simulink model "DC_drives_system"  (R2025b)
settings: Solver=FixedStepAuto  StartTime=0.0  StopTime=3.0  FixedStep=1e-4  RelTol=1e-3
values from neighbouring files (symbols this model uses):
  J_load = Simulink.Parameter    [dc_drives_system_parameter_declaraction.m]
  J_motor = Simulink.Parameter    [dc_drives_system_parameter_declaraction.m]    (also in motorised_BoB_system_with_PID.m)
  k_e = Simulink.Parameter    [dc_drives_system_parameter_declaraction.m]    (also in motorised_BoB_system_with_PID.m)
  k_t = Simulink.Parameter    [dc_drives_system_parameter_declaraction.m]    (also in motorised_BoB_system_with_PID.m)
  kFrs = Simulink.Parameter    [dc_drives_system_parameter_declaraction.m]    (also in motorised_BoB_system_with_PID.m)
  L_a = Simulink.Parameter    [dc_drives_system_parameter_declaraction.m]    (also in motorised_BoB_system_with_PID.m)
  R_a = Simulink.Parameter    [dc_drives_system_parameter_declaraction.m]    (also in motorised_BoB_system_with_PID.m)
  t_inv = Simulink.Parameter    [dc_drives_system_parameter_declaraction.m]    (also in motorised_BoB_system_with_PID.m)
  U_DC = Simulink.Parameter    [dc_drives_system_parameter_declaraction.m]    (also in motorised_BoB_system_with_PID.m)
  W_ci = Simulink.Parameter    [dc_drives_system_parameter_declaraction.m]    (also in motorised_BoB_system_with_PID.m)
  W_cq = Simulink.Parameter    [dc_drives_system_parameter_declaraction.m]    (also in motorised_BoB_system_with_PID.m)
  W_cw = Simulink.Parameter    [dc_drives_system_parameter_declaraction.m]    (also in motorised_BoB_system_with_PID.m)
undefined symbols (not defined in the file or in its folder): L, R
settings Model: Creator=fycce  LastModifiedBy=fycce

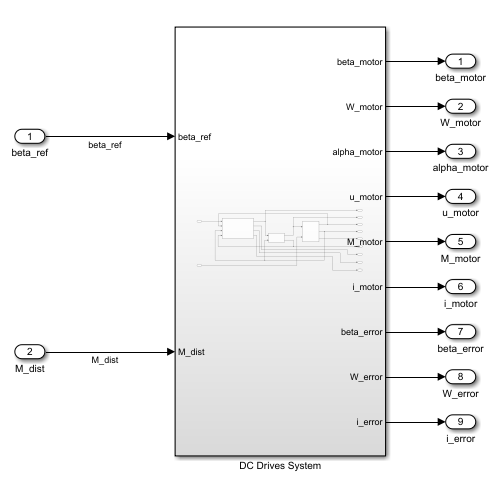
[thumbnail: Simulink's stored preview of the top-level diagram]
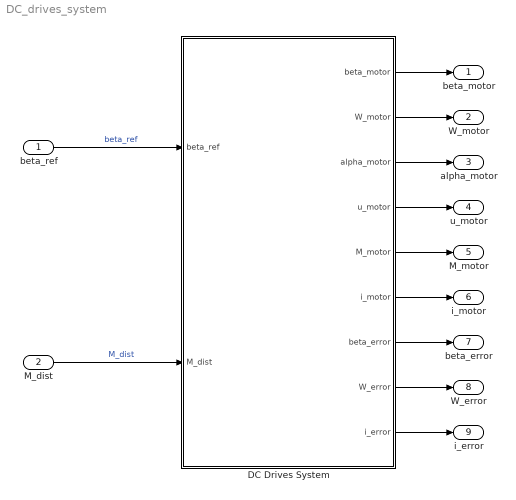
== system DC_drives_system ==
  beta_ref : Inport
  M_dist : Inport  Port=2
  DC Drives System : Subsystem
  beta_motor : Outport
  W_motor : Outport  Port=2
  alpha_motor : Outport  Port=3
  u_motor : Outport  Port=4
  M_motor : Outport  Port=5
  i_motor : Outport  Port=6
  beta_error : Outport  Port=7
  W_error : Outport  Port=8
  i_error : Outport  Port=9
  wires:
  DC Drives System/1(beta_motor) -> beta_motor/1
  DC Drives System/2(W_motor) -> W_motor/1
  DC Drives System/3(alpha_motor) -> alpha_motor/1
  DC Drives System/4(u_motor) -> u_motor/1
  DC Drives System/5(M_motor) -> M_motor/1
  DC Drives System/6(i_motor) -> i_motor/1
  DC Drives System/7(beta_error) -> beta_error/1
  DC Drives System/8(W_error) -> W_error/1
  DC Drives System/9(i_error) -> i_error/1
  M_dist/1 -> DC Drives System/2(M_dist)  "M_dist"
  beta_ref/1 -> DC Drives System/1(beta_ref)  "beta_ref"

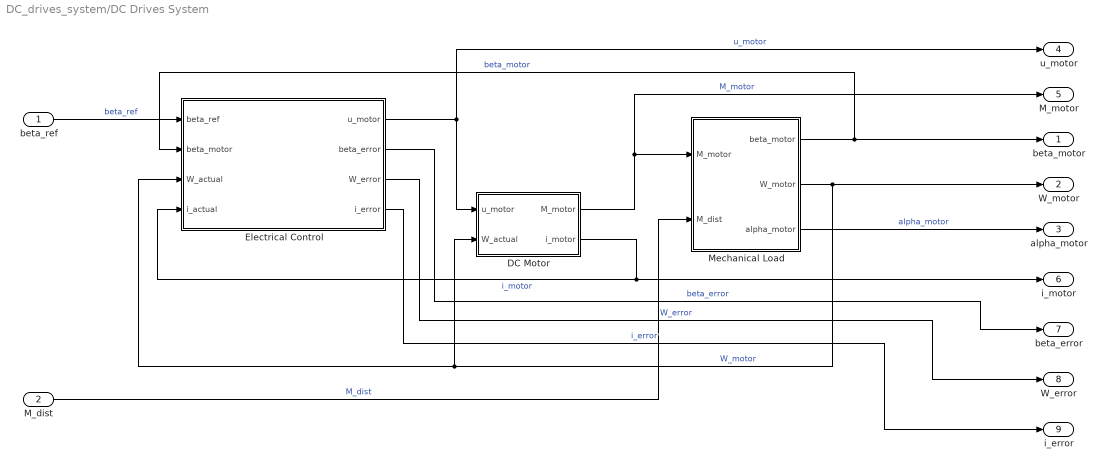
== system DC_drives_system/DC Drives System ==
  beta_ref : Inport
  M_dist : Inport  Port=2
  DC Motor : Subsystem
  Electrical Control : Subsystem
  Mechanical Load : Subsystem
  beta_motor : Outport
  W_motor : Outport  Port=2
  alpha_motor : Outport  Port=3
  u_motor : Outport  Port=4
  M_motor : Outport  Port=5
  i_motor : Outport  Port=6
  beta_error : Outport  Port=7
  W_error : Outport  Port=8
  i_error : Outport  Port=9
  wires:
  Electrical Control/2(beta_error) -> beta_error/1  "beta_error"
  Electrical Control/1(u_motor) -> u_motor/1, DC Motor/1(u_motor)  "u_motor"
  DC Motor/2(i_motor) -> Electrical Control/4(i_actual), i_motor/1  "i_motor"
  Mechanical Load/1(beta_motor) -> beta_motor/1, Electrical Control/2(beta_motor)  "beta_motor"
  Electrical Control/3(W_error) -> W_error/1  "W_error"
  beta_ref/1 -> Electrical Control/1(beta_ref)  "beta_ref"
  Mechanical Load/2(W_motor) -> W_motor/1, DC Motor/2(W_actual), Electrical Control/3(W_actual)  "W_motor"
  DC Motor/1(M_motor) -> M_motor/1, Mechanical Load/1(M_motor)  "M_motor"
  Electrical Control/4(i_error) -> i_error/1  "i_error"
  Mechanical Load/3(alpha_motor) -> alpha_motor/1  "alpha_motor"
  M_dist/1 -> Mechanical Load/2(M_dist)  "M_dist"

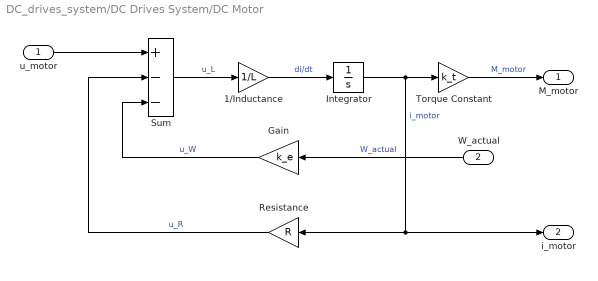
== system DC_drives_system/DC Drives System/DC Motor ==
  u_motor : Inport
  W_actual : Inport  Port=2
  1/Inductance : Gain  Gain=1/L
  Gain : Gain  Gain=k_e
  Integrator : Integrator
  Resistance : Gain  Gain=R
  Sum : Sum  Inputs=+--
  Torque Constant : Gain  Gain=k_t
  M_motor : Outport
  i_motor : Outport  Port=2
  wires:
  u_motor/1 -> Sum/1
  Sum/1 -> 1/Inductance/1  "u_L"
  1/Inductance/1 -> Integrator/1  "di/dt"
  Integrator/1 -> i_motor/1, Resistance/1, Torque Constant/1  "i_motor"
  Torque Constant/1 -> M_motor/1  "M_motor"
  Resistance/1 -> Sum/2  "u_R"
  Gain/1 -> Sum/3  "u_W"
  W_actual/1 -> Gain/1  "W_actual"

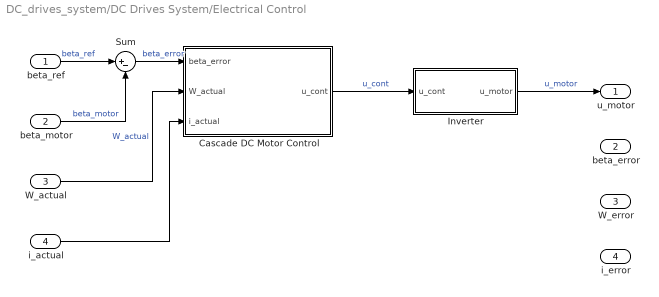
== system DC_drives_system/DC Drives System/Electrical Control ==
  beta_ref : Inport
  beta_motor : Inport  Port=2
  W_actual : Inport  Port=3
  i_actual : Inport  Port=4
  Cascade DC Motor Control : Subsystem
  Inverter : Subsystem
  Sum : Sum  Inputs=|+-
  u_motor : Outport
  beta_error : Outport  Port=2
  W_error : Outport  Port=3
  i_error : Outport  Port=4
  wires:
  Inverter/1(u_motor) -> u_motor/1  "u_motor"
  Cascade DC Motor Control/1(u_cont) -> Inverter/1(u_cont)  "u_cont"
  beta_ref/1 -> Sum/1  "beta_ref"
  beta_motor/1 -> Sum/2  "beta_motor"
  Sum/1 -> Cascade DC Motor Control/1(beta_error)  "beta_error"
  W_actual/1 -> Cascade DC Motor Control/2(W_actual)  "W_actual"
  i_actual/1 -> Cascade DC Motor Control/3(i_actual)

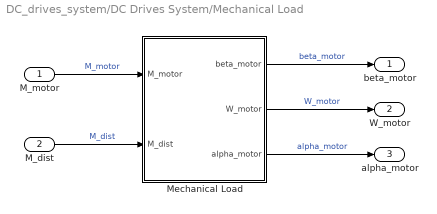
== system DC_drives_system/DC Drives System/Mechanical Load ==
  M_motor : Inport
  M_dist : Inport  Port=2
  Mechanical Load : Subsystem  Variant=on
  beta_motor : Outport
  W_motor : Outport  Port=2
  alpha_motor : Outport  Port=3
  wires:
  M_motor/1 -> Mechanical Load/1(M_motor)  "M_motor"
  Mechanical Load/2(W_motor) -> W_motor/1  "W_motor"
  Mechanical Load/1(beta_motor) -> beta_motor/1  "beta_motor"
  Mechanical Load/3(alpha_motor) -> alpha_motor/1  "alpha_motor"
  M_dist/1 -> Mechanical Load/2(M_dist)  "M_dist"

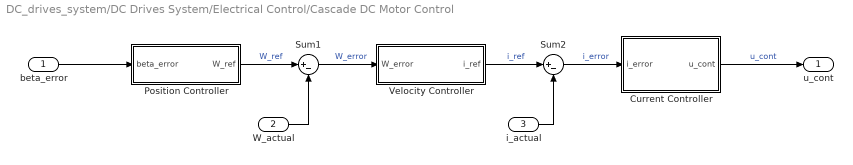
== system DC_drives_system/DC Drives System/Electrical Control/Cascade DC Motor Control ==
  beta_error : Inport
  W_actual : Inport  Port=2
  i_actual : Inport  Port=3
  Current Controller : Subsystem
  Position Controller : Subsystem
  Sum1 : Sum  Inputs=|+-
  Sum2 : Sum  Inputs=|+-
  Velocity Controller : Subsystem
  u_cont : Outport
  wires:
  Position Controller/1(W_ref) -> Sum1/1  "W_ref"
  Sum1/1 -> Velocity Controller/1(W_error)  "W_error"
  Velocity Controller/1(i_ref) -> Sum2/1  "i_ref"
  Sum2/1 -> Current Controller/1(i_error)  "i_error"
  beta_error/1 -> Position Controller/1(beta_error)
  Current Controller/1(u_cont) -> u_cont/1  "u_cont"
  i_actual/1 -> Sum2/2
  W_actual/1 -> Sum1/2

== system DC_drives_system/DC Drives System/Electrical Control/Inverter ==
  u_cont : Inport
  1st Order Lag : Subsystem
  U_DC Saturation : Saturate  UpperLimit=U_DC  LowerLimit=-U_DC
  u_motor : Outport
  wires:
  U_DC Saturation/1 -> u_motor/1  "u_motor"
  u_cont/1 -> 1st Order Lag/1(u_cont)  "u_cont"
  1st Order Lag/1(u_cont_lag) -> U_DC Saturation/1  "u_cont_lag"

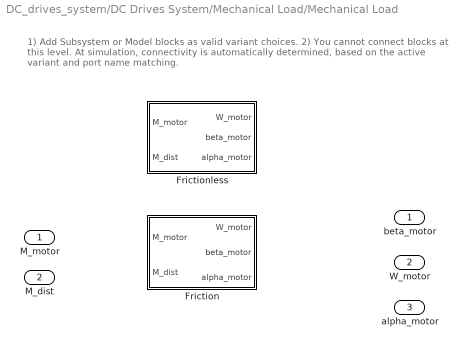
== system DC_drives_system/DC Drives System/Mechanical Load/Mechanical Load ==
  note: 1) Add Subsystem or Model blocks as valid variant choices.
      | 2) You cannot connect blocks at this level. At simulation, connectivity is automatically
      | determined, based on the active variant and port name matching.
  M_motor : Inport
  M_dist : Inport  Port=2
  Friction : Subsystem  VariantControl=choice == 1
  Frictionless : Subsystem  VariantControl=choice == 2
  beta_motor : Outport
  W_motor : Outport  Port=2
  alpha_motor : Outport  Port=3

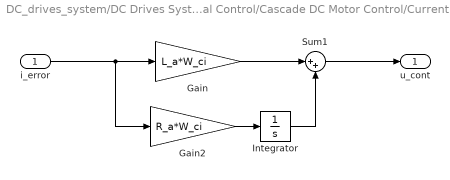
== system DC_drives_system/DC Drives System/Electrical Control/Cascade DC Motor Control/Current Controller ==
  i_error : Inport
  Gain : Gain  Gain=L_a*W_ci
  Gain2 : Gain  Gain=R_a*W_ci
  Integrator : Integrator
  Sum1 : Sum  Inputs=|++
  u_cont : Outport
  wires:
  Gain2/1 -> Integrator/1
  Gain/1 -> Sum1/1
  Integrator/1 -> Sum1/2
  i_error/1 -> Gain2/1, Gain/1
  Sum1/1 -> u_cont/1

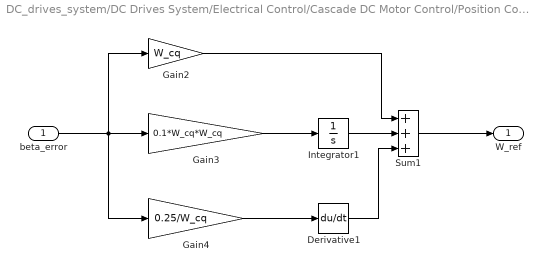
== system DC_drives_system/DC Drives System/Electrical Control/Cascade DC Motor Control/Position Controller ==
  beta_error : Inport
  Derivative1 : Derivative
  Gain2 : Gain  Gain=W_cq
  Gain3 : Gain  Gain=0.1*W_cq*W_cq
  Gain4 : Gain  Gain=0.25/W_cq
  Integrator1 : Integrator
  Sum1 : Sum  Inputs=+++
  W_ref : Outport
  wires:
  Sum1/1 -> W_ref/1
  beta_error/1 -> Gain3/1, Gain4/1, Gain2/1
  Gain2/1 -> Sum1/1
  Derivative1/1 -> Sum1/3
  Integrator1/1 -> Sum1/2
  Gain3/1 -> Integrator1/1
  Gain4/1 -> Derivative1/1

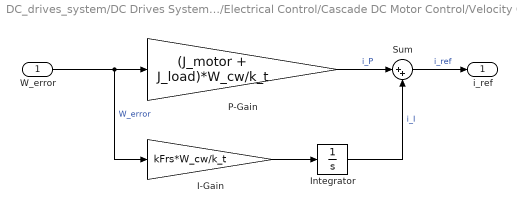
== system DC_drives_system/DC Drives System/Electrical Control/Cascade DC Motor Control/Velocity Controller ==
  W_error : Inport
  I-Gain : Gain  Gain=kFrs*W_cw/k_t
  Integrator : Integrator
  P-Gain : Gain  Gain=(J_motor + J_load)*W_cw/k_t
  Sum : Sum  Inputs=|++
  i_ref : Outport
  wires:
  W_error/1 -> I-Gain/1, P-Gain/1  "W_error"
  I-Gain/1 -> Integrator/1
  Sum/1 -> i_ref/1  "i_ref"
  P-Gain/1 -> Sum/1  "i_P"
  Integrator/1 -> Sum/2  "i_I"

== system DC_drives_system/DC Drives System/Electrical Control/Inverter/1st Order Lag ==
  u_cont : Inport
  Gain : Gain  Gain=1/t_inv
  Integrator : Integrator
  Sum : Sum  Inputs=|+-
  u_cont_lag : Outport
  wires:
  u_cont/1 -> Sum/1
  Sum/1 -> Gain/1
  Gain/1 -> Integrator/1
  Integrator/1 -> Sum/2, u_cont_lag/1

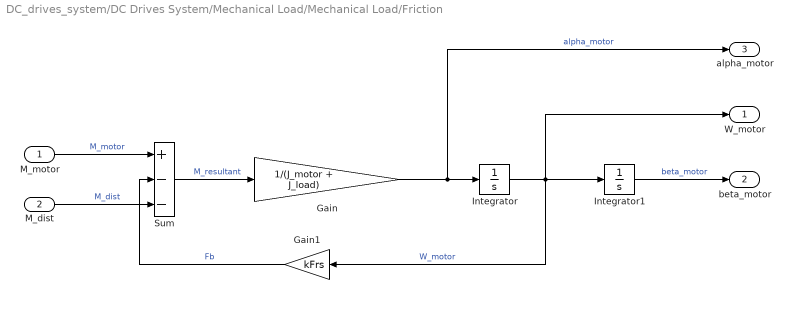
== system DC_drives_system/DC Drives System/Mechanical Load/Mechanical Load/Friction ==
  M_motor : Inport
  M_dist : Inport  Port=2
  Gain : Gain  Gain=1/(J_motor + J_load)
  Gain1 : Gain  Gain=kFrs
  Integrator : Integrator
  Integrator1 : Integrator
  Sum : Sum  Inputs=+--
  W_motor : Outport
  beta_motor : Outport  Port=2
  alpha_motor : Outport  Port=3
  wires:
  Integrator/1 -> Gain1/1, Integrator1/1, W_motor/1  "W_motor"
  Gain/1 -> Integrator/1, alpha_motor/1  "alpha_motor"
  Integrator1/1 -> beta_motor/1  "beta_motor"
  Sum/1 -> Gain/1  "M_resultant"
  M_motor/1 -> Sum/1  "M_motor"
  Gain1/1 -> Sum/2  "Fb"
  M_dist/1 -> Sum/3  "M_dist"

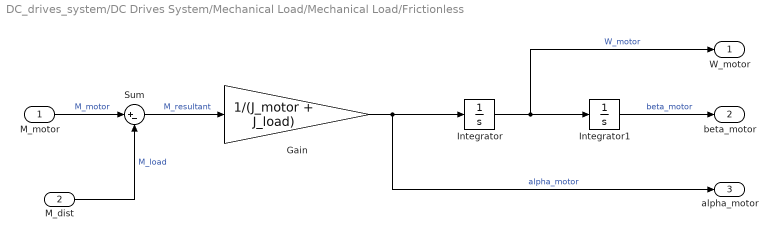
== system DC_drives_system/DC Drives System/Mechanical Load/Mechanical Load/Frictionless ==
  M_motor : Inport
  M_dist : Inport  Port=2
  Gain : Gain  Gain=1/(J_motor + J_load)
  Integrator : Integrator
  Integrator1 : Integrator
  Sum : Sum  Inputs=|+-
  W_motor : Outport
  beta_motor : Outport  Port=2
  alpha_motor : Outport  Port=3
  wires:
  Gain/1 -> Integrator/1, alpha_motor/1  "alpha_motor"
  Integrator/1 -> Integrator1/1, W_motor/1  "W_motor"
  Integrator1/1 -> beta_motor/1  "beta_motor"
  M_motor/1 -> Sum/1  "M_motor"
  M_dist/1 -> Sum/2  "M_load"
  Sum/1 -> Gain/1  "M_resultant"
